simulink model "example_EnergyTapping"  (R2018b)
settings: Solver=ode45  StartTime=0.0  StopTime=24*3600  MaxStep=60  RelTol=1e-3  EnableMultiTasking=on
libraries: carnot x7
settings Model: Creator=drhf  LastModifiedBy=drhf
settings DataIOCC: LimitDataPoints=on  SaveFormat=Array  SignalLoggingSaveFormat=ModelDataLogs
settings OptimizationCC: ExpressionDepthLimit=2147483647  LifeSpan=inf
settings DebuggingCC: UnderspecifiedInitializationDetection=Classic  MergeDetectMultiDrivingBlocksExec=none  SolverPrmCheckMsg=warning  FcnCallInpInsideContextMsg=warning  StateNameClashWarn=warning  SFUnexpectedBacktrackingDiag=warning  SFNoUnconditionalDefaultTransitionDiag=warning  SFExecutionAtInitializationDiag=none
settings HardwareCC: ProdBitPerPointer=32  ProdBitPerSizeT=32  ProdBitPerPtrDiffT=32  ProdLargestAtomicFloat=None  ProdIntDivRoundTo=Undefined  ProdEndianess=Unspecified  ProdWordSize=32  ProdHWDeviceType=32-bit Generic
settings ModelReferenceCC: PropagateSignalLabelsOutOfModel=off
settings SFSimCC: SimUseLocalCustomCode=off
settings RTWCC: RTWUseLocalCustomCode=off
settings CodeAppCC: StateflowObjectComments=on
settings GRTTargetCC: TargetLangStandard=C89/C90 (ANSI)  GeneratePreprocessorConditionals=Disable all  CombineOutputUpdateFcns=off  GRTInterface=on
settings ConfigComp: CovMetricSettings=dw  CovHtmlReporting=on  CovSaveCumulativeToWorkspaceVar=on  CovSaveSingleToWorkspaceVar=on  CovExternalEMLEnable=off

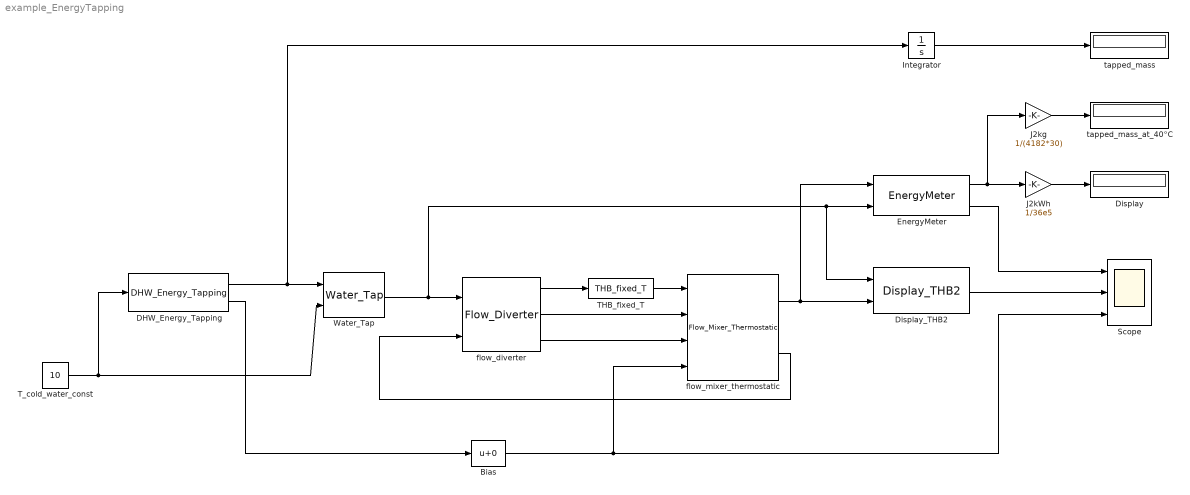
== system example_EnergyTapping ==
  Bias : Bias
  DHW_Energy_Tapping : carnot/Load/Hot_Water_Tapping/DHW_Energy_Tapping  mdot_nom=1/60  times="[7     7.1 7.5   8.083 8.25  8.5   8.75  9     9.5   10.5  11.5  11.75 12.75 14.5  15.5  16.5  18    18.25 18.5  19    20.5  21.25 21.5]*3600"  energies=[0.105 1.4 0.105 0.105 0.105 0.105 0.105 0.105 0.105 0.105 0.105 0.105 0.315 0.105 0.105 0.105 0.105 0.105 0.105 0.105 0.735 0.105 1.4 ]*36e5  dT_set="[30    30  30    30    30    30    30    30    30    30    30    30    45    30    30    30    30    30    30    30    45    30    30  ]"  coeffs="[3     6   3     3     3     3     3     3     3     3     3     3     4     3     3     3     3     3     3     3     4     3     6   ]"
      settings: SourceProductName=Carnot
  Display : Display
  Display_THB2 : carnot/Outputs/Display_THB2  t=off  m=on  p=off  id=off  mix=off  d=off
      settings: SourceProductName=Carnot
  EnergyMeter : carnot/Control/EnergyMeter
      settings: SourceProductName=Carnot
  Integrator : Integrator
  J2kWh : Gain  Gain=1/36e5
  J2kg : Gain  Gain=1/(4182*30)
  Scope : Scope  NumInputPorts=3
  THB_fixed_T : carnot/Source/Simple/THB_fixed_T  t=60
      settings: SourceProductName=Carnot
  T_cold_water_const : Constant  Value=10
  Water_Tap : carnot/Load/Hot_Water_Tapping/Water_Tap  dia=0.02  p=2e5
      settings: SourceProductName=Carnot
  flow_diverter : carnot/Hydraulics/Flow_Diverter
      settings: SourceProductName=Carnot
  flow_mixer_thermostatic : carnot/Hydraulics/Flow_Mixer_Thermostatic  t=10
      settings: SourceProductName=Carnot
  tapped_mass : Display
  tapped_mass_at_40°C : Display
  wires:
  flow_diverter/3 -> flow_mixer_thermostatic/3
  flow_diverter/2 -> flow_mixer_thermostatic/2
  THB_fixed_T/1 -> flow_mixer_thermostatic/1
  flow_mixer_thermostatic/2 -> flow_diverter/2
  T_cold_water_const/1 -> Water_Tap/2, DHW_Energy_Tapping/1
  flow_diverter/1 -> THB_fixed_T/1
  Integrator/1 -> tapped_mass/1
  J2kg/1 -> tapped_mass_at_40°C/1
  EnergyMeter/1 -> J2kg/1, J2kWh/1
  Water_Tap/1 -> EnergyMeter/2, Display_THB2/1, flow_diverter/1
  flow_mixer_thermostatic/1 -> Display_THB2/2, EnergyMeter/1
  DHW_Energy_Tapping/2 -> Bias/1
  Display_THB2/1 -> Scope/2
  DHW_Energy_Tapping/1 -> Integrator/1, Water_Tap/1
  J2kWh/1 -> Display/1
  EnergyMeter/2 -> Scope/1
  Bias/1 -> Scope/3, flow_mixer_thermostatic/4
